simulink model "MilTesting"  (R2020b)
settings: Solver=VariableStepAuto  StartTime=0.0  StopTime=10.0  RelTol=1e-3
undefined symbols (not defined in the file or in its folder): sigbuilder_block
settings Model: Creator=99003778  LastModifiedBy=99003778

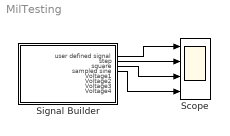
== system MilTesting ==
  Scope : Scope  NumInputPorts=4
  Signal Builder : Subsystem  Tag=STV Subsys  LoadFcn=sigbuilder_block('load');  StartFcn=sigbuilder_block('start');  StopFcn=sigbuilder_block('stop');  ClipboardFcn=sigbuilder_block('clipboard');  mask(Sigbuilder block){tuvar=[0:10]}
      mask help: Simulink:masks:SigbuilderBlock_MD
      mask init:
      | if ~strcmp(get_param(bdroot(gcbh),'SimulationStatus'),'stopped') tuvar = sigbuilder_block('maskInit'); end
      settings: CopyFcn=sigbuilder_block('copy');  DeleteFcn=sigbuilder_block('delete');  ModelCloseFcn=sigbuilder_block('modelClose');  PreSaveFcn=sigbuilder_block('preSave');  PauseFcn=sigbuilder_block('pause');  ContinueFcn=sigbuilder_block('continue');  NameChangeFcn=sigbuilder_block('namechange');  OpenFcn=sigbuilder_block('open',[6 30 948 639.75 ]);  CloseFcn=sigbuilder_block('close');
      mask Display: plot(0, 0, 100, 100,[2, 2, 32, 32, 2], [68, 8, 8, 68, 68],[32, 2], [38, 38], [32, 19, 2],[53, 60, 44], [32, 17, 17, 2],[16, 16, 31, 31]);txt = getActiveGroup(gcbh);text(2, 100, txt,'verticalAlignment', 'top');
  wires:
  Signal Builder/2(step) -> Scope/2
  Signal Builder/1(user defined signal) -> Scope/1
  Signal Builder/3(square) -> Scope/3
  Signal Builder/4(sampled sine) -> Scope/4

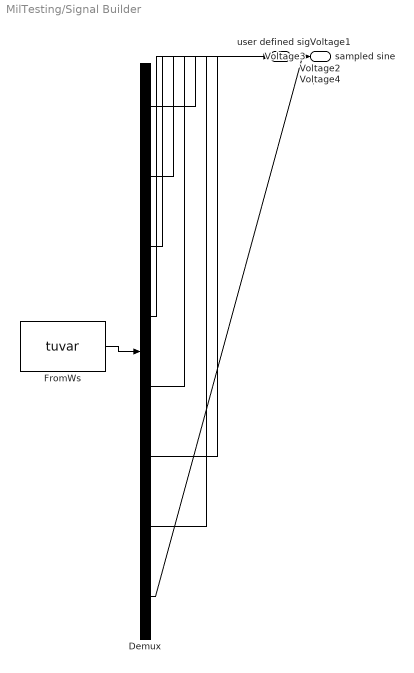
== system MilTesting/Signal Builder ==
  Demux : Demux  Tag=STV Demux  Outputs=8
      settings: DisplayOption=none
  FromWs : FromWorkspace  Tag=STV FromWs  VariableName=tuvar
      SigBuilderData=|
      | common.afterFinalStr = 'Extrapolate'
      | common.sampleTime = 0
      | dataSet.timeRange = [0 10]
      | dataSet.name = 'Group 1'
      | sbobj.Groups.Name = 'Group 1'
      | sbobj.Groups.Signals(1).Name = 'user defined signal'
      | sbobj.Groups.Signals(1).XData = [0 4 4 4.9 4.9 5.4 5.4 6 6 10]
      | sbobj.Groups.Signals(1).YData = [0 0 1 0.9955 0.995 0.995 0.993 0.99 0 0]
      | sbobj.Groups.Signals(2).Name = 'step'
      | sbobj.Groups.Signals(2).XData = [0 5 5 10]
      | sbobj.Groups.Signals(2).YData = [0 0 1 1]
      | sbobj.Groups.Signals(3).Name = 'square'
      | sbobj.Groups.Signals(3).XData = [0 4 4 6 6 10]
      | sbobj.Groups.Signals(3).YData = [0 0 1 1 0 0]
      | sbobj.Groups.Signals(4).Name = 'sampled sine'
      | sbobj.Groups.Signals(4).XData = [0 0.125 0.25 0.375 0.5 0.625 0.75 0.875 1 1.125 1.25 1.375 1.5 1.625 1.75 1.875 2 2.125 2.25 2.375 2.5 2.625 2.75 2.875 3 3.125 3.25 3.375 3.5 3.625 3.75 3.875 4 4.125 4.25 4.375 4.5 4.625 4.75 4.875 5 5.125 5.25 5.375 5.5 5.625 5.75 5.875 6 6.125 6.25 6.375 6.5 6.625 6.75 6.875 7 7.125 7.25 7.375 7.5 7.625 7.75 7.875 8 8.125 8.25 8.375 8.5 8.625 8.75 8.875 9 9.125 9.25 9.375 9.5 9.625 9.75 9.875 10]
      | sbobj.Groups.Signals(4).YData = [1 1.70710678119 2 1.70710678119 1 0.292893218813 0 0.292893218813 1 1.70710678119 2 1.70710678119 1 0.292893218813 0 0.292893218813 1 1.70710678119 2 1.70710678119 1 0.292893218813 0 0.292893218813 1 1.70710678119 2 1.70710678119 1 0.292893218813 0 0.292893218813 1 1.70710678119 2 1.70710678119 1 0.292893218813 0 0.292893218813 1 1.70710678119 2 1.70710678119 1 0.292893218813 0 0.292893218813 1 1.70710678119 2 1.70710678119 1 0.292893218813 0 0.292893218813 1 1.70710678119 2 1.70710678119 1 0.292893218813 0 0.292893218813 1 1.70710678119 2 1.70710678119 1 0.292893218813 0 0.292893218813 1 1.70710678119 2 1.70710678119 1 0.292893218813 0 0.292893218813 1]
      | sbobj.Groups.Signals(5).Name = 'Voltage1'
      | sbobj.Groups.Signals(5).XData = [0 0.1 0.2 0.3 0.4 0.5 0.6 0.7 0.8 0.9 1 1.1 1.2 10]
      | sbobj.Groups.Signals(5).YData = [10 20 30 40 50 60 70 80 90 100 110 120 130 130]
      | sbobj.Groups.Signals(6).Name = 'Voltage2'
      | sbobj.Groups.Signals(6).XData = [0 0.1 0.2 0.3 0.4 0.5 0.6 0.7 0.8 0.9 1 1.1 1.2 10]
      | sbobj.Groups.Signals(6).YData = [9 6 4 6 2 8 6 9 2 5 1 8 0 0]
      | sbobj.Groups.Signals(7).Name = 'Voltage3'
      | sbobj.Groups.Signals(7).XData = [0 1 2 3 4 5 6 7 8 9 10 11 12]
      | sbobj.Groups.Signals(7).YData = [10 20 30 40 50 60 70 80 90 100 110 120 130]
      | sbobj.Groups.Signals(8).Name = 'Voltage4'
      | sbobj.Groups.Signals(8).XData = [0 1 2 3 4 5 6 7 8 9 10 11 12]
      | sbobj.Groups.Signals(8).YData = [9 6 4 6 2 8 6 9 2 5 1 8 0]
  user defined signal : Outport  Tag=STV Outport
  step : Outport  Tag=STV Outport  Port=2
  square : Outport  Tag=STV Outport  Port=3
  sampled sine : Outport  Tag=STV Outport  Port=4
  Voltage1 : Outport  Tag=STV Outport  Port=5
  Voltage2 : Outport  Tag=STV Outport  Port=6
  Voltage3 : Outport  Tag=STV Outport  Port=7
  Voltage4 : Outport  Tag=STV Outport  Port=8
  wires:
  Demux/1 -> user defined signal/1
  FromWs/1 -> Demux/1
  Demux/2 -> step/1
  Demux/3 -> square/1
  Demux/4 -> sampled sine/1
  Demux/5 -> Voltage1/1
  Demux/6 -> Voltage2/1
  Demux/7 -> Voltage3/1
  Demux/8 -> Voltage4/1
